simulink model "microMouseSimulator"  (R2019b)
settings: Solver=ode4  StartTime=0.0  StopTime=EndTime  FixedStep=Simulation_Step  MinStep=0.1  RelTol=1e-3
undefined symbols (not defined in the file): theta0, x0, y0
settings Model: Creator=r720r  LastModifiedBy=r720r
settings DataIOCC: SaveOutput=off  SignalLogging=off  DSMLogging=off  SaveTime=off  ReturnWorkspaceOutputs=off

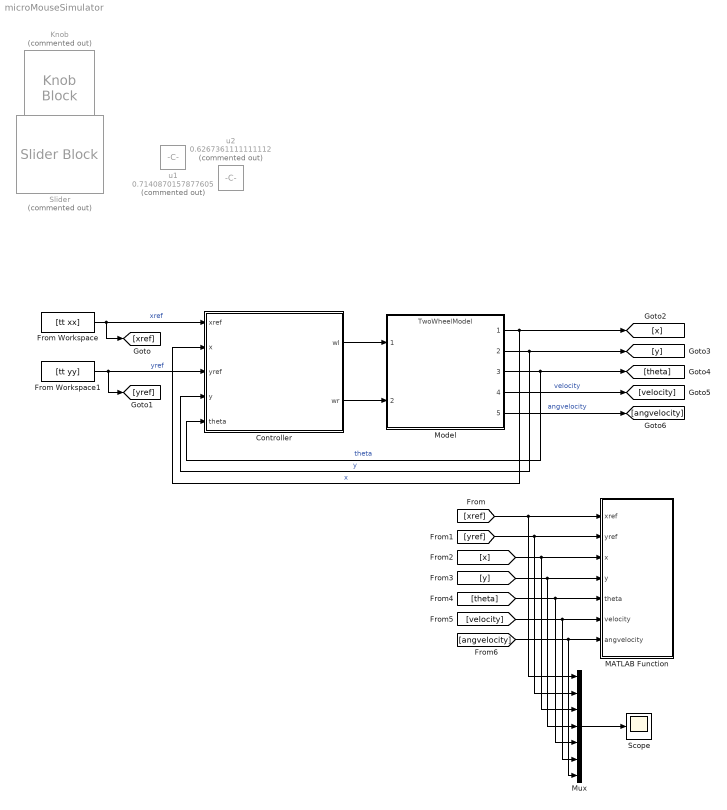
== system microMouseSimulator ==
  Controller : Subsystem
  From Workspace : FromWorkspace  VariableName=[tt xx]  SampleTime=0  Interpolate=off  OutputAfterFinalValue=Holding final value
  From Workspace1 : FromWorkspace  VariableName=[tt yy]  SampleTime=0  Interpolate=off  OutputAfterFinalValue=Holding final value
  Knob : KnobBlock  Commented=on  ScaleMax=1
  MATLAB Function : MATLAB Function  TreatAsAtomicUnit=on
  Model : ModelReference  ModelNameDialog=TwoWheelModel.slx  ModelReferenceVersion=1.10
  Mux : Mux  Inputs=7
  Scope : Scope
  Slider : SliderBlock  Commented=on  ScaleMin=-2  ScaleMax=2  TickInterval=1
  u1 : Constant  Commented=on  Value=0.7140870157877605
  u2 : Constant  Commented=on  Value=0.6267361111111112
  wires:
  Model/1 -> Controller/2(x), [x]  "x"
  Model/2 -> Controller/4(y), [y]  "y"
  Model/3 -> Controller/5(theta), [theta]  "theta"
  Model/4 -> [velocity]  "velocity"
  Model/5 -> [angvelocity]  "angvelocity"
  From Workspace/1 -> [xref], Controller/1(xref)  "xref"
  From Workspace1/1 -> [yref], Controller/3(yref)  "yref"
  Controller/1(wl) -> Model/1
  Controller/2(wr) -> Model/2
  [x] -> Mux/3, MATLAB Function/3(x)
  [y] -> Mux/4, MATLAB Function/4(y)
  [theta] -> Mux/5, MATLAB Function/5(theta)
  [velocity] -> Mux/6, MATLAB Function/6(velocity)
  [angvelocity] -> Mux/7, MATLAB Function/7(angvelocity)
  [xref] -> Mux/1, MATLAB Function/1(xref)
  [yref] -> Mux/2, MATLAB Function/2(yref)
  Mux/1 -> Scope/1

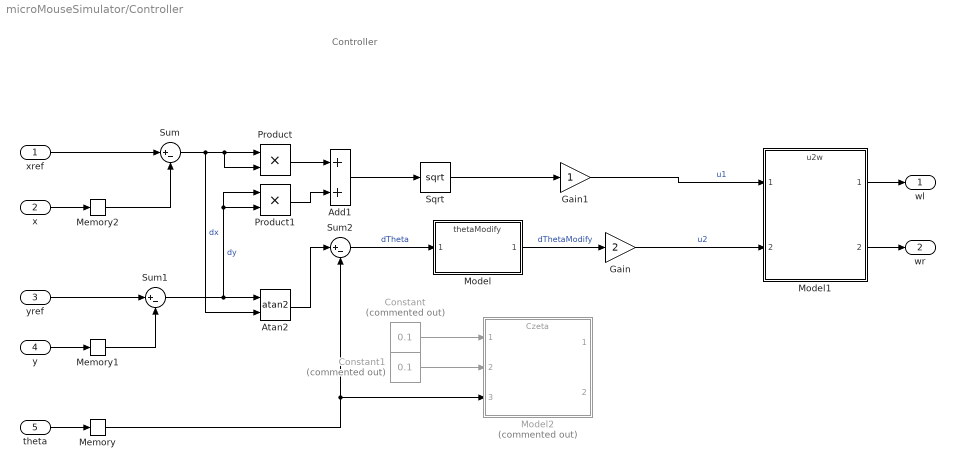
== system microMouseSimulator/Controller ==
  note: Controller
  xref : Inport
  x : Inport  Port=2
  yref : Inport  Port=3
  y : Inport  Port=4
  theta : Inport  Port=5
  Add1 : Sum
  Atan2 : Trigonometry  Operator=atan2
  Constant : Constant  Commented=on  Value=0.1
  Constant1 : Constant  Commented=on  Value=0.1
  Gain : Gain  Gain=2
  Gain1 : Gain
  Memory : Memory  InitialCondition=theta0  InheritSampleTime=on
  Memory1 : Memory  InitialCondition=y0  InheritSampleTime=on
  Memory2 : Memory  InitialCondition=x0  InheritSampleTime=on
  Model : ModelReference  ModelNameDialog=thetaModify.slx  ModelReferenceVersion=1.4
  Model1 : ModelReference  ModelNameDialog=u2w.slx  ModelReferenceVersion=1.3
  Model2 : ModelReference  Commented=on  ModelNameDialog=Czeta.slx  ModelReferenceVersion=1.5
  Product : Product
  Product1 : Product
  Sqrt : Sqrt  SaturateOnIntegerOverflow=on
  Sum : Sum  Inputs=|+-
  Sum1 : Sum  Inputs=|+-
  Sum2 : Sum  Inputs=|+-
  wl : Outport
  wr : Outport  Port=2
  wires:
  Model1/1 -> wl/1
  Memory1/1 -> Sum1/2
  Sqrt/1 -> Gain1/1
  Model1/2 -> wr/1
  x/1 -> Memory2/1
  yref/1 -> Sum1/1
  theta/1 -> Memory/1
  xref/1 -> Sum/1
  y/1 -> Memory1/1
  Memory2/1 -> Sum/2
  Product/1 -> Add1/1
  Add1/1 -> Sqrt/1
  Product1/1 -> Add1/2
  Atan2/1 -> Sum2/1
  Memory/1 -> Model2/3, Sum2/2
  Sum/1 -> Product/1, Product/2, Atan2/2  "dx"
  Sum1/1 -> Product1/1, Product1/2, Atan2/1  "dy"
  Sum2/1 -> Model/1  "dTheta"
  Model/1 -> Gain/1  "dThetaModify"
  Constant/1 -> Model2/1
  Constant1/1 -> Model2/2
  Gain1/1 -> Model1/1  "u1"
  Gain/1 -> Model1/2  "u2"

== matlab function microMouseSimulator/MATLAB Function ==
  data: xref input; yref input; x input; y input; theta input; velocity input; angvelocity input
function fcn(xref, yref, x, y, theta, velocity, angvelocity)
    coder.extrinsic('evalin', 'plot', 'setfield', 'redraw');
    TwoWheel = evalin('base','TwoWheel'); 
    %fig = evalin('base','fig'); %ベースワークスペースのハンドル取得
    
    hXYrefPoint = evalin('base','hXYrefPoint');
    set(hXYrefPoint,'xdata',xref,'ydata',yref);
    
    TwoWheel = setfield(TwoWheel, 'X', x);
    TwoWheel = setfield(TwoWheel, 'Y', y);
    TwoWheel = setfield(TwoWheel, 'Theta', theta);
    TwoWheel = setfield(TwoWheel, 'Velocity', velocity);
    TwoWheel = setfield(TwoWheel, 'AngVelocity', angvelocity);
    
    redraw(TwoWheel);
    %set はグラフィックス オブジェクトのプロパティの設定
